simulink model "model_report_gutman_lqr2"  (R2018b)
settings: Solver=FixedStepAuto  StartTime=0.0  StopTime=10  FixedStep=Ts/100  RelTol=1e-3
StopFcn:
  | %figure;plot(true_position.Data(:,1),true_position.Data(:,2))
values from neighbouring files (symbols this model uses):
  b = 1.115    [report_gutman.m]
  bike_params = [g h b a lambda m]    [report_gutman.m]
  complementary = 0.985    [report_gutman.m]
  g = 9.81    [report_gutman.m]
  IMU_height = 0.45    [report_gutman.m]
  initial_roll = deg2rad(2)    [report_gutman.m]
  initial_rollrate = deg2rad(2)    [report_gutman.m]
  lambda = deg2rad(90-24)    [report_gutman.m]
  num_tf_steering = [253.4]    [report_gutman.m]
  Ts = 0.01    [report_gutman.m]
  v = 4    [report_gutman.m]
undefined symbols (not defined in the file or in its folder): A, B, C, D, lqr_gains, Ts_IMU, velocity_lqr
libraries: simulink_extras x8
settings Model: Creator=maximef  LastModifiedBy=maximef

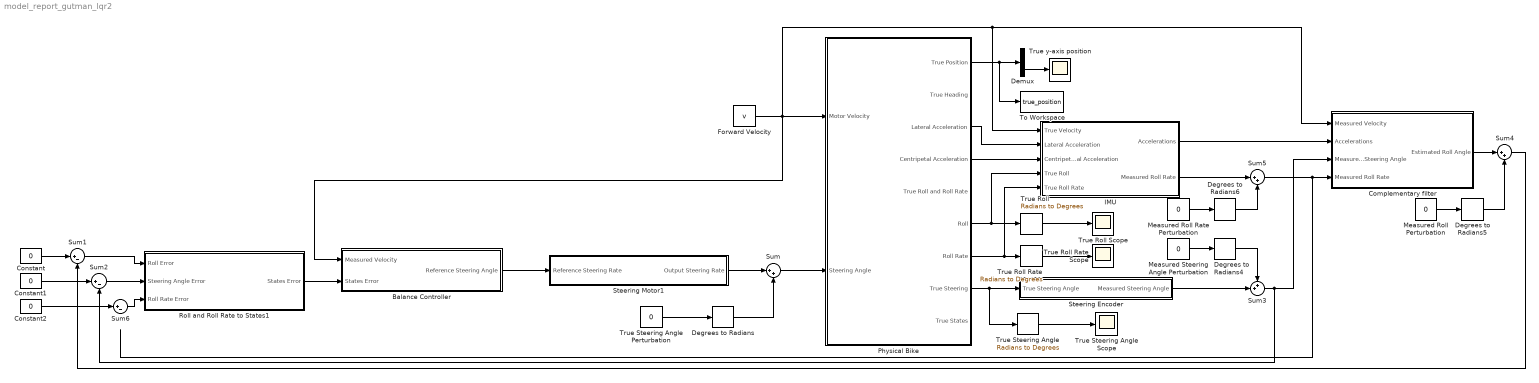
== system model_report_gutman_lqr2 ==
  Balance Controller : Subsystem  SystemSampleTime=Ts
  Complementary filter : Subsystem  SystemSampleTime=Ts_IMU
  Constant : Constant  Value=0
  Constant1 : Constant  Value=0
  Constant2 : Constant  Value=0
  Degrees to Radians{,4..6} (4 alike) : simulink_extras/Transformations/Degrees to Radians
  Demux : Demux  Outputs=2
  Forward Velocity : Constant  Value=v
  IMU : Subsystem  TreatAsAtomicUnit=on
  Measured Roll Perturbation : Constant  Value=0
  Measured Roll Rate Perturbation : Constant  Value=0
  Measured Steering Angle Perturbation : Constant  Value=0
  Physical Bike : Subsystem
  Roll and Roll Rate to States1 : Subsystem
  Steering Encoder : Subsystem  TreatAsAtomicUnit=on  SystemSampleTime=Ts
  Steering Motor1 : Subsystem
  Sum : Sum  Inputs=|++
  Sum1 : Sum  Inputs=|+-
  Sum2 : Sum  Inputs=|+-
  Sum3 : Sum  Inputs=++|
  Sum4 : Sum  Inputs=|++
  Sum5 : Sum  Inputs=|++
  Sum6 : Sum  Inputs=|+-
  To Workspace : ToWorkspace  VariableName=true_position  SaveFormat=Timeseries  SampleTime=Ts
  True Roll : simulink_extras/Transformations/Radians to Degrees
  True Roll Rate : simulink_extras/Transformations/Radians to Degrees
  True Roll Rate Scope : Scope
  True Roll Scope : Scope
  True Steering Angle : simulink_extras/Transformations/Radians to Degrees
  True Steering Angle Perturbation : Constant  Value=0
  True Steering Angle Scope : Scope
  True y-axis position : Scope
  wires:
  True Roll Rate/1 -> True Roll Rate Scope/1
  Physical Bike/3(Lateral Acceleration) -> IMU/2(Lateral Acceleration)
  Physical Bike/7(Roll Rate) -> IMU/5(True Roll Rate), True Roll Rate/1
  Measured Roll Rate Perturbation/1 -> Degrees to Radians6/1
  Physical Bike/6(Roll) -> IMU/4(True Roll), True Roll/1
  Sum/1 -> Physical Bike/2(Steering Angle)
  Measured Steering Angle Perturbation/1 -> Degrees to Radians4/1
  True Steering Angle/1 -> True Steering Angle Scope/1
  Physical Bike/4(Centripetal Acceleration) -> IMU/3(Centripetal Acceleration)
  IMU/1(Accelerations) -> Complementary filter/2(Accelerations)
  Sum3/1 -> Sum2/2, Complementary filter/3(Measured Steering Angle)
  True Steering Angle Perturbation/1 -> Degrees to Radians/1
  Measured Roll Perturbation/1 -> Degrees to Radians5/1
  Forward Velocity/1 -> Complementary filter/1(Measured Velocity), IMU/1(True Velocity), Balance Controller/1(Measured Velocity), Physical Bike/1(Motor Velocity)
  Degrees to Radians/1 -> Sum/2
  Balance Controller/1(Reference Steering Angle) -> Steering Motor1/1(Reference Steering Rate)
  True Roll/1 -> True Roll Scope/1
  Steering Encoder/1(Measured Steering Angle) -> Sum3/2
  Degrees to Radians6/1 -> Sum5/2
  Degrees to Radians4/1 -> Sum3/1
  Physical Bike/8(True Steering) -> True Steering Angle/1, Steering Encoder/1(True Steering Angle)
  IMU/2(Measured Roll Rate) -> Sum5/1
  Sum4/1 -> Sum1/2
  Sum5/1 -> Complementary filter/4("Measured Roll Rate ")
  Physical Bike/1(True Position) -> To Workspace/1, Demux/1
  Demux/2 -> True y-axis position/1
  Steering Motor1/1(Output Steering Rate) -> Sum/1
  Roll and Roll Rate to States1/1(States Error) -> Balance Controller/2(States Error)
  Sum1/1 -> Roll and Roll Rate to States1/1(Roll Error)
  Sum6/1 -> Roll and Roll Rate to States1/3(Roll Rate Error)
  Sum2/1 -> Roll and Roll Rate to States1/2(Steering Angle Error)
  Constant/1 -> Sum1/1
  Constant1/1 -> Sum2/1
  Constant2/1 -> Sum6/1
  Degrees to Radians5/1 -> Sum4/2
  Complementary filter/1(Estimated Roll Angle) -> Sum4/1

== system model_report_gutman_lqr2/Balance Controller ==
  Measured Velocity : Inport
  States Error : Inport  Port=2
  LQR Controller : Subsystem  TreatAsAtomicUnit=on  SystemSampleTime=Ts
  Reference Steering Angle : Outport
  wires:
  States Error/1 -> LQR Controller/2(State Error)
  LQR Controller/1(Calculated Input) -> Reference Steering Angle/1
  Measured Velocity/1 -> LQR Controller/1(Velocity)

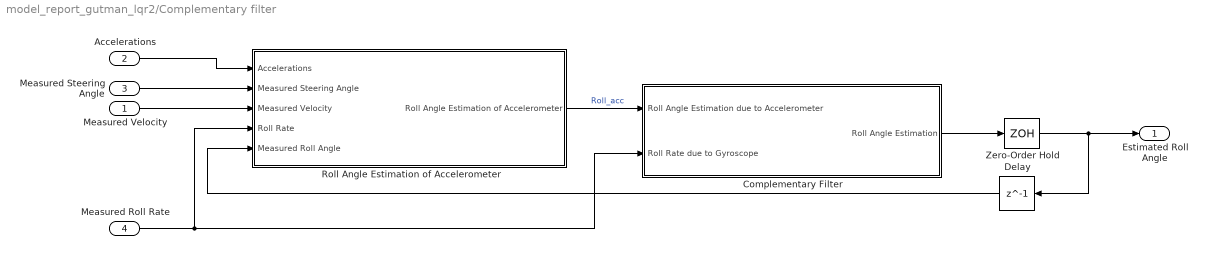
== system model_report_gutman_lqr2/Complementary filter ==
  Measured Velocity : Inport
  Accelerations : Inport  Port=2
  Measured Steering Angle : Inport  Port=3
  "Measured Roll Rate " : Inport  Port=4
  Complementary Filter : Subsystem  TreatAsAtomicUnit=on  SystemSampleTime=Ts
  Delay : Delay  DelayLength=1
  Roll Angle Estimation of Accelerometer : Subsystem
  Zero-Order Hold : ZeroOrderHold  SampleTime=Ts
  Estimated Roll Angle : Outport
  wires:
  Roll Angle Estimation of Accelerometer/1(Roll Angle Estimation of Accelerometer) -> Complementary Filter/1(Roll Angle Estimation due to Accelerometer)  "Roll_acc"
  Delay/1 -> Roll Angle Estimation of Accelerometer/5(Measured Roll Angle)
  Measured Velocity/1 -> Roll Angle Estimation of Accelerometer/3(Measured Velocity)
  Measured Steering Angle/1 -> Roll Angle Estimation of Accelerometer/2(Measured Steering Angle)
  "Measured Roll Rate "/1 -> Complementary Filter/2(Roll Rate due to Gyroscope), Roll Angle Estimation of Accelerometer/4(Roll Rate)
  Accelerations/1 -> Roll Angle Estimation of Accelerometer/1(Accelerations)
  Complementary Filter/1(Roll Angle Estimation) -> Zero-Order Hold/1
  Zero-Order Hold/1 -> Estimated Roll Angle/1, Delay/1

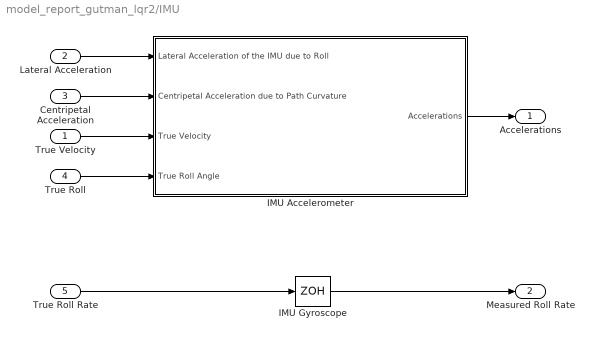
== system model_report_gutman_lqr2/IMU ==
  True Velocity : Inport
  Lateral Acceleration : Inport  Port=2
  Centripetal Acceleration : Inport  Port=3
  True Roll : Inport  Port=4
  True Roll Rate : Inport  Port=5
  IMU Accelerometer : Subsystem
  IMU Gyroscope : ZeroOrderHold  SampleTime=-1
  Accelerations : Outport
  Measured Roll Rate : Outport  Port=2
  wires:
  True Velocity/1 -> IMU Accelerometer/3(True Velocity)
  Lateral Acceleration/1 -> IMU Accelerometer/1(Lateral Acceleration of the IMU due to Roll)
  Centripetal Acceleration/1 -> IMU Accelerometer/2(Centripetal Acceleration due to Path Curvature)
  True Roll/1 -> IMU Accelerometer/4(True Roll Angle)
  IMU Accelerometer/1(Accelerations) -> Accelerations/1
  IMU Gyroscope/1 -> Measured Roll Rate/1
  True Roll Rate/1 -> IMU Gyroscope/1

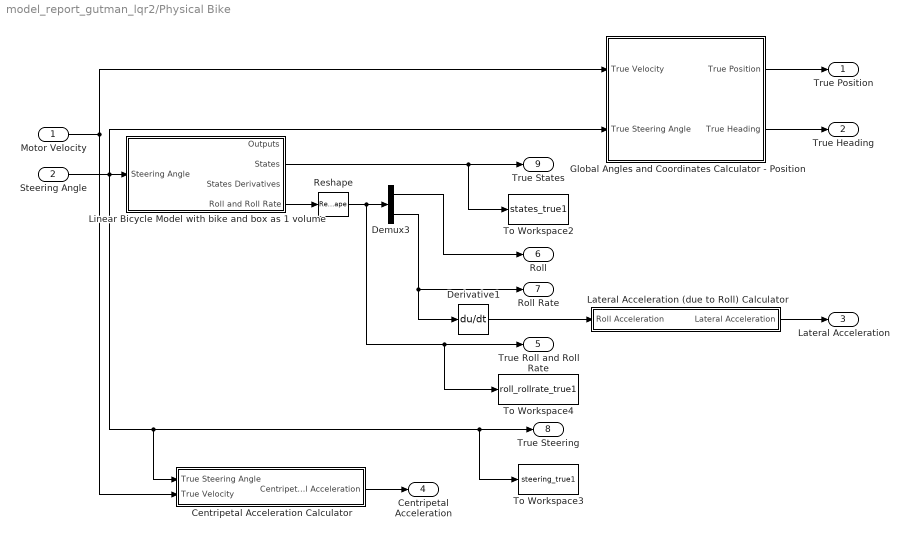
== system model_report_gutman_lqr2/Physical Bike ==
  Motor Velocity : Inport
  Steering Angle : Inport  Port=2
  Centripetal Acceleration Calculator : Subsystem
  Demux3 : Demux  Outputs=2
  Derivative1 : Derivative  CoefficientInTFapproximation=Inf
  Global Angles and Coordinates Calculator - Position : Subsystem  SystemSampleTime=Ts
  Lateral Acceleration (due to Roll) Calculator : Subsystem
  Linear Bicycle Model with bike and box as 1 volume : Subsystem
  Reshape : Reshape
  To Workspace2 : ToWorkspace  VariableName=states_true1  SaveFormat=Timeseries  SampleTime=-1
  To Workspace3 : ToWorkspace  VariableName=steering_true1  SaveFormat=Timeseries  SampleTime=-1
  To Workspace4 : ToWorkspace  VariableName=roll_rollrate_true1  SaveFormat=Timeseries  SampleTime=-1
  True Position : Outport
  True Heading : Outport  Port=2
  Lateral Acceleration : Outport  Port=3
  Centripetal Acceleration : Outport  Port=4
  True Roll and Roll Rate : Outport  Port=5
  Roll : Outport  Port=6
  Roll Rate : Outport  Port=7
  True Steering : Outport  Port=8
  True States : Outport  Port=9
  wires:
  Steering Angle/1 -> Global Angles and Coordinates Calculator - Position/2(True Steering Angle), To Workspace3/1, True Steering/1, Centripetal Acceleration Calculator/1(True Steering Angle), Linear Bicycle Model with bike and box as 1 volume/1(Steering Angle)
  Centripetal Acceleration Calculator/1(Centripetal Acceleration) -> Centripetal Acceleration/1
  Derivative1/1 -> Lateral Acceleration (due to Roll) Calculator/1(Roll Acceleration)
  Lateral Acceleration (due to Roll) Calculator/1(Lateral Acceleration) -> Lateral Acceleration/1
  Demux3/2 -> Derivative1/1, Roll Rate/1
  Linear Bicycle Model with bike and box as 1 volume/2(States) -> To Workspace2/1, True States/1
  Demux3/1 -> Roll/1
  Reshape/1 -> To Workspace4/1, True Roll and Roll Rate/1, Demux3/1
  Linear Bicycle Model with bike and box as 1 volume/4(Roll and Roll Rate) -> Reshape/1
  Motor Velocity/1 -> Centripetal Acceleration Calculator/2(True Velocity), Global Angles and Coordinates Calculator - Position/1(True Velocity)
  Global Angles and Coordinates Calculator - Position/1(True Position) -> True Position/1
  Global Angles and Coordinates Calculator - Position/2(True Heading) -> True Heading/1

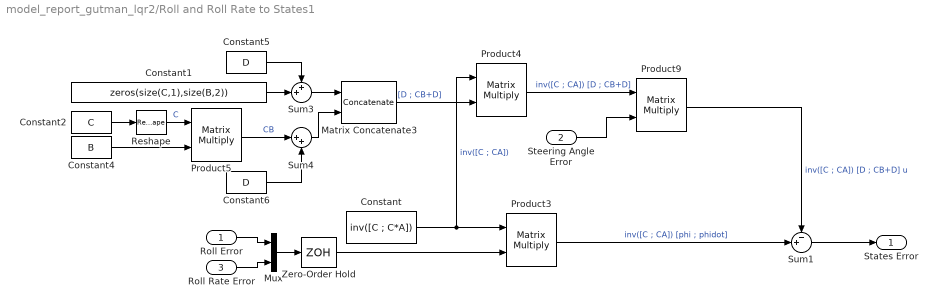
== system model_report_gutman_lqr2/Roll and Roll Rate to States1 ==
  Roll Error : Inport
  Steering Angle Error : Inport  Port=2
  Roll Rate Error : Inport  Port=3
  Constant : Constant  Value=inv([C ; C*A])
  Constant1 : Constant  Value=zeros(size(C,1),size(B,2))
  Constant2 : Constant  Value=C
  Constant4 : Constant  Value=B
  Constant5 : Constant  Value=D
  Constant6 : Constant  Value=D
  Matrix Concatenate3 : Concatenate  Mode=Multidimensional array
  Mux : Mux  Inputs=2
  Product{3..5,9} (4 alike) : Product  SCDEnableBlockLinearizationSpecification=on  Multiplication=Matrix(*)
  Reshape : Reshape  OutputDimensionality=Customize  OutputDimensions=[size(C,1),size(C,2)]
  Sum1 : Sum  Inputs=-+|
  Sum3 : Sum  Inputs=++|
  Sum4 : Sum  Inputs=|++
  Zero-Order Hold : ZeroOrderHold  SampleTime=Ts
  States Error : Outport
  wires:
  Constant2/1 -> Reshape/1
  Constant/1 -> Product4/1, Product3/1  "inv([C ; CA])"
  Mux/1 -> Zero-Order Hold/1
  Product3/1 -> Sum1/2  "inv([C ; CA]) [phi ; phidot]"
  Matrix Concatenate3/1 -> Product4/2  "[D ; CB+D]"
  Product5/1 -> Sum4/1  "CB"
  Constant4/1 -> Product5/2
  Constant1/1 -> Sum3/2
  Product4/1 -> Product9/1  "inv([C ; CA]) [D ; CB+D]"
  Steering Angle Error/1 -> Product9/2
  Product9/1 -> Sum1/1  "inv([C ; CA]) [D ; CB+D] u"
  Sum1/1 -> States Error/1
  Zero-Order Hold/1 -> Product3/2
  Constant6/1 -> Sum4/2
  Constant5/1 -> Sum3/1
  Sum4/1 -> Matrix Concatenate3/2
  Sum3/1 -> Matrix Concatenate3/1
  Reshape/1 -> Product5/1  "C"
  Roll Error/1 -> Mux/1
  Roll Rate Error/1 -> Mux/2

== system model_report_gutman_lqr2/Steering Encoder ==
  True Steering Angle : Inport
  Zero-Order Hold : ZeroOrderHold  SampleTime=Ts
  Measured Steering Angle : Outport
  wires:
  True Steering Angle/1 -> Zero-Order Hold/1
  Zero-Order Hold/1 -> Measured Steering Angle/1

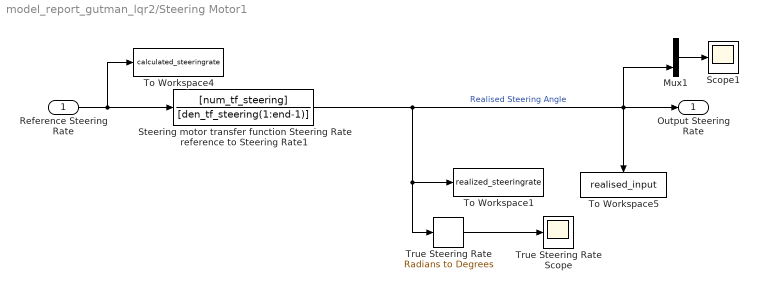
== system model_report_gutman_lqr2/Steering Motor1 ==
  Reference Steering Rate : Inport
  Mux1 : Mux  Inputs=2
  Scope1 : Scope
  Steering motor transfer function Steering Rate reference to Steering Rate1 : TransferFcn  Numerator=[num_tf_steering]  Denominator=[den_tf_steering(1:end-1)]
  To Workspace1 : ToWorkspace  VariableName=realized_steeringrate  SaveFormat=Timeseries  SampleTime=Ts
  To Workspace4 : ToWorkspace  VariableName=calculated_steeringrate  SaveFormat=Timeseries  SampleTime=Ts
  To Workspace5 : ToWorkspace  VariableName=realised_input  SaveFormat=Timeseries  SampleTime=Ts
  True Steering Rate : simulink_extras/Transformations/Radians to Degrees
  True Steering Rate Scope : Scope
  Output Steering Rate : Outport
  wires:
  Mux1/1 -> Scope1/1
  Steering motor transfer function Steering Rate reference to Steering Rate1/1 -> Output Steering Rate/1, Mux1/2, To Workspace5/1, True Steering Rate/1, To Workspace1/1  "Realised Steering Angle"
  True Steering Rate/1 -> True Steering Rate Scope/1
  Reference Steering Rate/1 -> To Workspace4/1, Steering motor transfer function Steering Rate reference to Steering Rate1/1

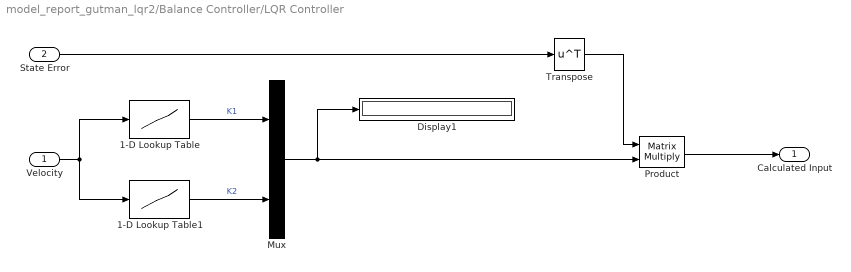
== system model_report_gutman_lqr2/Balance Controller/LQR Controller ==
  Velocity : Inport
  State Error : Inport  Port=2
  1-D Lookup Table : Lookup_n-D  NumberOfTableDimensions=1  BreakpointsForDimension1=velocity_lqr  BreakpointsForDimension2=velocity_lqr  BreakpointsForDimension3=velocity_lqr  BreakpointsForDimension4=velocity_lqr  Table=lqr_gains(:,2)  InternalRulePriority=Speed  RndMeth=Simplest  InputSameDT=on
  1-D Lookup Table1 : Lookup_n-D  NumberOfTableDimensions=1  BreakpointsForDimension1=velocity_lqr  BreakpointsForDimension2=velocity_lqr  BreakpointsForDimension3=velocity_lqr  BreakpointsForDimension4=velocity_lqr  Table=lqr_gains(:,3)  InternalRulePriority=Speed  RndMeth=Simplest  InputSameDT=on
  Display1 : Display
  Mux : Mux  Inputs=2
  Product : Product  Multiplication=Matrix(*)
  Transpose : Math  Operator=transpose  SaturateOnIntegerOverflow=on
  Calculated Input : Outport
  wires:
  1-D Lookup Table/1 -> Mux/1  "K1"
  1-D Lookup Table1/1 -> Mux/2  "K2"
  Velocity/1 -> 1-D Lookup Table1/1, 1-D Lookup Table/1
  Mux/1 -> Product/2, Display1/1
  Transpose/1 -> Product/1
  Product/1 -> Calculated Input/1
  State Error/1 -> Transpose/1

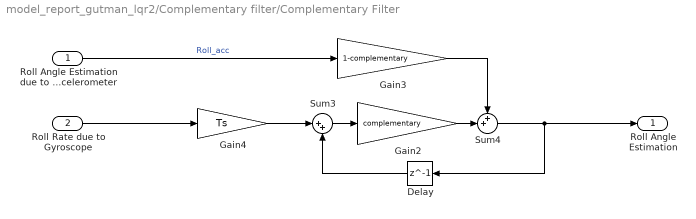
== system model_report_gutman_lqr2/Complementary filter/Complementary Filter ==
  Roll Angle Estimation due to Accelerometer : Inport
  Roll Rate due to Gyroscope : Inport  Port=2
  Delay : Delay  DelayLength=1  InitialCondition=initial_roll
  Gain2 : Gain  Gain=complementary
  Gain3 : Gain  Gain=1-complementary
  Gain4 : Gain  Gain=Ts
  Sum3 : Sum  Inputs=|++
  Sum4 : Sum  Inputs=++|
  Roll Angle Estimation : Outport
  wires:
  Roll Angle Estimation due to Accelerometer/1 -> Gain3/1  "Roll_acc"
  Sum3/1 -> Gain2/1
  Roll Rate due to Gyroscope/1 -> Gain4/1
  Delay/1 -> Sum3/2
  Gain4/1 -> Sum3/1
  Gain2/1 -> Sum4/2
  Gain3/1 -> Sum4/1
  Sum4/1 -> Delay/1, Roll Angle Estimation/1

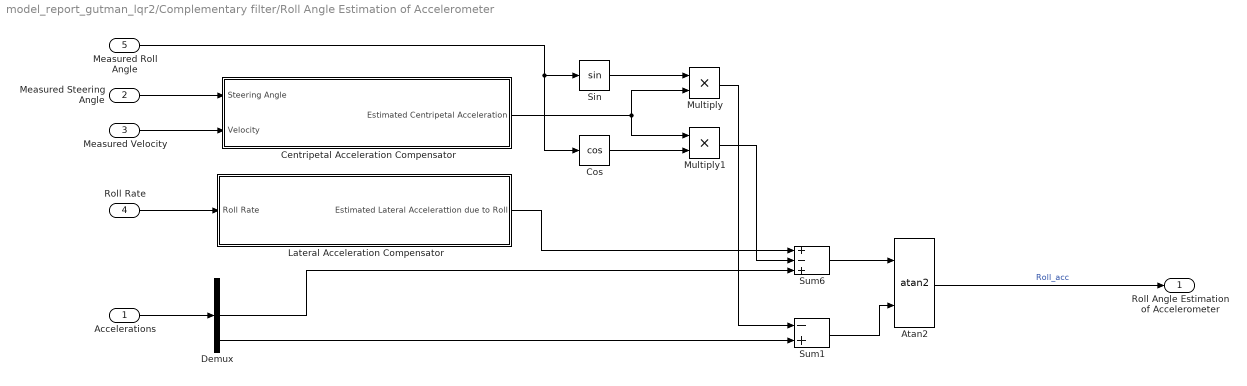
== system model_report_gutman_lqr2/Complementary filter/Roll Angle Estimation of Accelerometer ==
  Accelerations : Inport
  Measured Steering Angle : Inport  Port=2
  Measured Velocity : Inport  Port=3
  Roll Rate : Inport  Port=4
  Measured Roll Angle : Inport  Port=5
  Atan2 : Trigonometry  Operator=atan2
  Centripetal Acceleration Compensator : Subsystem
  Cos : Trigonometry  Operator=cos
  Demux : Demux  Outputs=3
  Lateral Acceleration Compensator : Subsystem
  Multiply : Product
  Multiply1 : Product
  Sin : Trigonometry
  Sum1 : Sum  Inputs=-+
  Sum6 : Sum  Inputs=+-+
  Roll Angle Estimation of Accelerometer : Outport
  wires:
  Sum1/1 -> Atan2/2
  Lateral Acceleration Compensator/1(Estimated Lateral Accelerattion due to Roll) -> Sum6/1
  Atan2/1 -> Roll Angle Estimation of Accelerometer/1  "Roll_acc"
  Roll Rate/1 -> Lateral Acceleration Compensator/1(Roll Rate)
  Accelerations/1 -> Demux/1
  Measured Velocity/1 -> Centripetal Acceleration Compensator/2(Velocity)
  Measured Steering Angle/1 -> Centripetal Acceleration Compensator/1(Steering Angle)
  Centripetal Acceleration Compensator/1(Estimated Centripetal Acceleration) -> Multiply/2, Multiply1/1
  Measured Roll Angle/1 -> Sin/1, Cos/1
  Cos/1 -> Multiply1/2
  Sin/1 -> Multiply/1
  Multiply1/1 -> Sum6/2
  Demux/3 -> Sum1/2
  Multiply/1 -> Sum1/1
  Sum6/1 -> Atan2/1
  Demux/2 -> Sum6/3

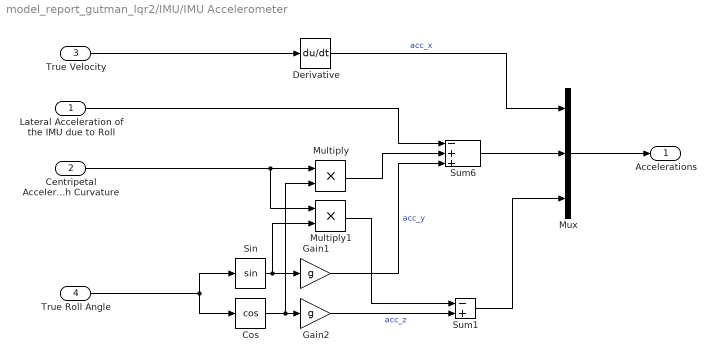
== system model_report_gutman_lqr2/IMU/IMU Accelerometer ==
  Lateral Acceleration of the IMU due to Roll : Inport
  Centripetal Acceleration due to Path Curvature : Inport  Port=2
  True Velocity : Inport  Port=3
  True Roll Angle : Inport  Port=4
  Cos : Trigonometry  Operator=cos
  Derivative : Derivative  CoefficientInTFapproximation=-1
  Gain1 : Gain  Gain=g
  Gain2 : Gain  Gain=g
  Multiply : Product
  Multiply1 : Product
  Mux : Mux  Inputs=3
  Sin : Trigonometry
  Sum1 : Sum  Inputs=-+
  Sum6 : Sum  Inputs=-++
  Accelerations : Outport
  wires:
  Multiply/1 -> Sum6/2
  Gain1/1 -> Sum6/3  "acc_y"
  Sin/1 -> Multiply1/2, Gain1/1
  Derivative/1 -> Mux/1  "acc_x"
  Cos/1 -> Multiply/2, Gain2/1
  Gain2/1 -> Sum1/2  "acc_z"
  True Roll Angle/1 -> Sin/1, Cos/1
  True Velocity/1 -> Derivative/1
  Centripetal Acceleration due to Path Curvature/1 -> Multiply1/1, Multiply/1
  Multiply1/1 -> Sum1/1
  Sum1/1 -> Mux/3
  Mux/1 -> Accelerations/1
  Sum6/1 -> Mux/2
  Lateral Acceleration of the IMU due to Roll/1 -> Sum6/1

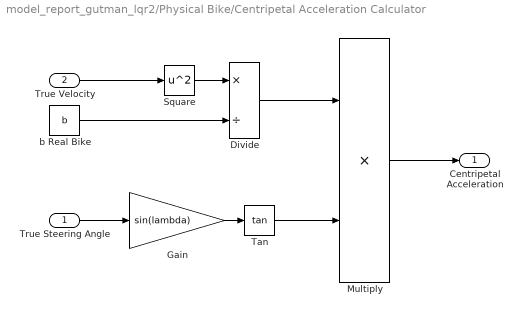
== system model_report_gutman_lqr2/Physical Bike/Centripetal Acceleration Calculator ==
  True Steering Angle : Inport
  True Velocity : Inport  Port=2
  Divide : Product  Inputs=*/
  Gain : Gain  Gain=sin(lambda)
  Multiply : Product
  Square : Math  Operator=square  SaturateOnIntegerOverflow=on
  Tan : Trigonometry  Operator=tan
  b Real Bike : Constant  Value=b
  Centripetal Acceleration : Outport
  wires:
  True Velocity/1 -> Square/1
  Square/1 -> Divide/1
  b Real Bike/1 -> Divide/2
  True Steering Angle/1 -> Gain/1
  Divide/1 -> Multiply/1
  Tan/1 -> Multiply/2
  Multiply/1 -> Centripetal Acceleration/1
  Gain/1 -> Tan/1

== system model_report_gutman_lqr2/Physical Bike/Global Angles and Coordinates Calculator - Position ==
  note: True Steering
      | Angle
  True Velocity : Inport
  True Steering Angle : Inport  Port=2
  Gain1 : Gain  Gain=sin(lambda)
  Measured Bike Angles to Global Angles : Subsystem
  Measured Global Angles to Global Coordinates : Subsystem
  Sum : Sum  Inputs=++|
  True Position : Outport
  True Heading : Outport  Port=2
  wires:
  Measured Bike Angles to Global Angles/1(Psi) -> Sum/2, Measured Global Angles to Global Coordinates/2(Psi)
  Gain1/1 -> Measured Bike Angles to Global Angles/2(Measured Steering Angle)
  Sum/1 -> True Heading/1
  Measured Bike Angles to Global Angles/2(Beta) -> Sum/1, Measured Global Angles to Global Coordinates/3(Beta)
  Measured Global Angles to Global Coordinates/1("Position (X, Y)") -> True Position/1
  True Velocity/1 -> Measured Global Angles to Global Coordinates/1(Velocity), Measured Bike Angles to Global Angles/1(Velocity)
  True Steering Angle/1 -> Gain1/1

== system model_report_gutman_lqr2/Physical Bike/Lateral Acceleration (due to Roll) Calculator ==
  Roll Acceleration : Inport
  Constant3 : Constant  Value=IMU_height
  Multiply : Product
  Lateral Acceleration : Outport
  wires:
  Multiply/1 -> Lateral Acceleration/1
  Constant3/1 -> Multiply/1
  Roll Acceleration/1 -> Multiply/2

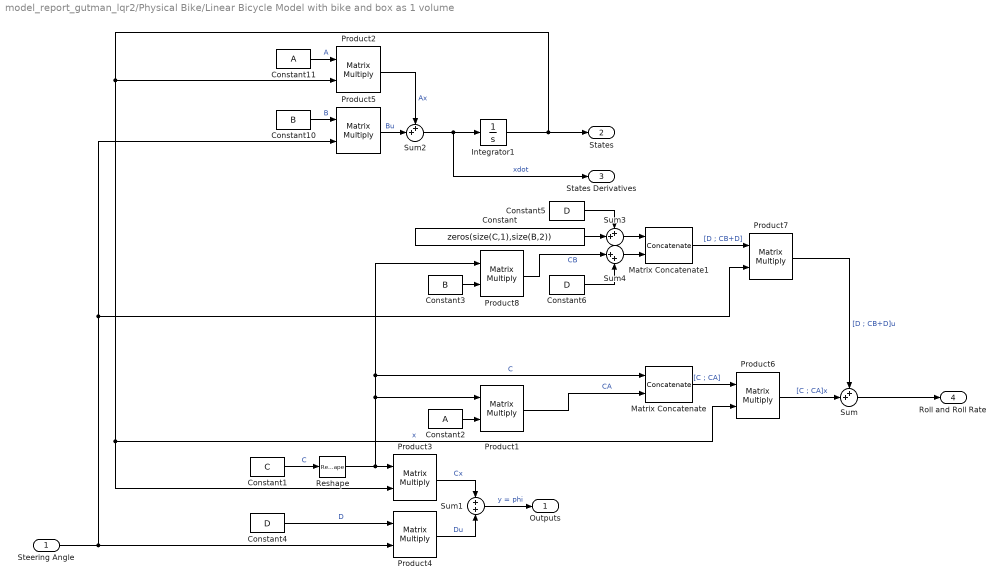
== system model_report_gutman_lqr2/Physical Bike/Linear Bicycle Model with bike and box as 1 volume ==
  Steering Angle : Inport
  Constant : Constant  Value=zeros(size(C,1),size(B,2))
  Constant1 : Constant  Value=C
  Constant10 : Constant  Value=B
  Constant11 : Constant  Value=A
  Constant2 : Constant  Value=A
  Constant3 : Constant  Value=B
  Constant4 : Constant  Value=D
  Constant5 : Constant  Value=D
  Constant6 : Constant  Value=D
  Integrator1 : Integrator  InitialCondition=[C ; C*A]\[initial_roll ; initial_rollrate]
  Matrix Concatenate : Concatenate  Mode=Multidimensional array
  Matrix Concatenate1 : Concatenate  Mode=Multidimensional array
  Product{1..8} (8 alike) : Product  SCDEnableBlockLinearizationSpecification=on  Multiplication=Matrix(*)
  Reshape : Reshape  OutputDimensionality=Customize  OutputDimensions=[size(C,1),size(C,2)]
  Sum : Sum  Inputs=++|
  Sum1 : Sum
  Sum2 : Sum  Inputs=++|
  Sum3 : Sum  Inputs=++|
  Sum4 : Sum  Inputs=|++
  Outputs : Outport
  States : Outport  Port=2
  States Derivatives : Outport  Port=3
  Roll and Roll Rate : Outport  Port=4
  wires:
  Reshape/1 -> Product3/1, Product8/1, Matrix Concatenate/1, Product1/1  "C"
  Sum/1 -> Roll and Roll Rate/1
  Constant1/1 -> Reshape/1  "C"
  Matrix Concatenate/1 -> Product6/1  "[C ; CA]"
  Product5/1 -> Sum2/2  "Bu"
  Matrix Concatenate1/1 -> Product7/1  "[D ; CB+D]"
  Constant11/1 -> Product2/1  "A"
  Constant3/1 -> Product8/2
  Product6/1 -> Sum/2  "[C ; CA]x"
  Sum2/1 -> Integrator1/1, States Derivatives/1  "xdot"
  Product2/1 -> Sum2/1  "Ax"
  Product1/1 -> Matrix Concatenate/2  "CA"
  Product8/1 -> Sum4/1  "CB"
  Integrator1/1 -> Product2/2, Product6/2, Product3/2, States/1  "x"
  Sum1/1 -> Outputs/1  "y = phi"
  Constant2/1 -> Product1/2
  Product7/1 -> Sum/1  "[D ; CB+D]u"
  Constant10/1 -> Product5/1  "B"
  Steering Angle/1 -> Product4/2, Product5/2, Product7/2
  Product4/1 -> Sum1/2  "Du"
  Product3/1 -> Sum1/1  "Cx"
  Constant4/1 -> Product4/1  "D"
  Sum3/1 -> Matrix Concatenate1/1
  Constant/1 -> Sum3/2
  Constant5/1 -> Sum3/1
  Sum4/1 -> Matrix Concatenate1/2
  Constant6/1 -> Sum4/2

== system model_report_gutman_lqr2/Complementary filter/Roll Angle Estimation of Accelerometer/Centripetal Acceleration Compensator ==
  Steering Angle : Inport
  Velocity : Inport  Port=2
  Bike Model b : Constant  Value=b
  Divide : Product  Inputs=*/
  Gain : Gain  Gain=sin(lambda)
  Multiply : Product
  Square : Math  Operator=square  SaturateOnIntegerOverflow=on
  Tan : Trigonometry  Operator=tan
  Estimated Centripetal Acceleration : Outport
  wires:
  Velocity/1 -> Square/1
  Square/1 -> Divide/1
  Bike Model b/1 -> Divide/2
  Steering Angle/1 -> Gain/1
  Divide/1 -> Multiply/1
  Tan/1 -> Multiply/2
  Multiply/1 -> Estimated Centripetal Acceleration/1
  Gain/1 -> Tan/1

== system model_report_gutman_lqr2/Complementary filter/Roll Angle Estimation of Accelerometer/Lateral Acceleration Compensator ==
  Roll Rate : Inport
  Constant4 : Constant  Value=IMU_height
  Multiply1 : Product
  Numerical Derivative : Subsystem
  Estimated Lateral Accelerattion due to Roll : Outport
  wires:
  Numerical Derivative/1(Roll Acceleration) -> Multiply1/2  "roll angular acceleration"
  Constant4/1 -> Multiply1/1
  Multiply1/1 -> Estimated Lateral Accelerattion due to Roll/1  "lateral acceleration"
  Roll Rate/1 -> Numerical Derivative/1(Roll Rate)

== system model_report_gutman_lqr2/Physical Bike/Global Angles and Coordinates Calculator - Position/Measured Bike Angles to Global Angles ==
  Velocity : Inport
  Measured Steering Angle : Inport  Port=2
  " Bike Parameters Model " : Constant  Value=bike_params
  Integrator : Integrator
  MATLAB Function : MATLAB Function  TreatAsAtomicUnit=on
  Psi : Outport
  Beta : Outport  Port=2
  wires:
  MATLAB Function/2(beta) -> Beta/1
  MATLAB Function/1(psi_d) -> Integrator/1
  Integrator/1 -> Psi/1
  " Bike Parameters Model "/1 -> MATLAB Function/2(bike_params)
  Measured Steering Angle/1 -> MATLAB Function/3(delta)
  Velocity/1 -> MATLAB Function/1(v)

== system model_report_gutman_lqr2/Physical Bike/Global Angles and Coordinates Calculator - Position/Measured Global Angles to Global Coordinates ==
  Velocity : Inport
  Psi : Inport  Port=2
  Beta : Inport  Port=3
  Integrator1 : Integrator
  Integrator2 : Integrator
  MATLAB Function1 : MATLAB Function  TreatAsAtomicUnit=on
  Mux : Mux  Inputs=2
  "Position (X, Y)" : Outport
  wires:
  MATLAB Function1/2(Ydot) -> Integrator2/1  "Ydot"
  MATLAB Function1/1(Xdot) -> Integrator1/1  "Xdot"
  Psi/1 -> MATLAB Function1/2(psi)
  Beta/1 -> MATLAB Function1/3(beta)
  Velocity/1 -> MATLAB Function1/1(v)
  Integrator2/1 -> Mux/2
  Integrator1/1 -> Mux/1
  Mux/1 -> "Position (X, Y)"/1

== system model_report_gutman_lqr2/Complementary filter/Roll Angle Estimation of Accelerometer/Lateral Acceleration Compensator/Numerical Derivative ==
  Roll Rate : Inport
  Delay18 : Delay  DelayLength=1
  Gain3 : Gain  Gain=1/Ts
  Sum3 : Sum  Inputs=|+-
  Roll Acceleration : Outport
  wires:
  Sum3/1 -> Gain3/1
  Delay18/1 -> Sum3/2
  Roll Rate/1 -> Sum3/1, Delay18/1
  Gain3/1 -> Roll Acceleration/1

== matlab function model_report_gutman_lqr2/Physical Bike/Global Angles and Coordinates Calculator - Position/Measured Bike Angles to Global Angles/MATLAB Function ==
  data: v input; bike_params input; delta input; psi_d output; beta output
function [psi_d, beta]  = fcn(v, bike_params, delta)

b = bike_params(3);
a = bike_params(4);

beta = atan((a / (b)) * tan(delta));
psi_d = (v / a) * sin(beta);

== matlab function model_report_gutman_lqr2/Physical Bike/Global Angles and Coordinates Calculator - Position/Measured Global Angles to Global Coordinates/MATLAB Function1 ==
  data: v input; psi input; Xdot output; beta input; Ydot output
function [Xdot, Ydot]  = fcn(v, psi, beta)

Xdot = v * cos(psi + beta);
Ydot = v * sin(psi + beta);
